simulink model "Digitizing_3delays_1us_pi_wPi2"  (R2014a)
settings: Solver=FixedStepDiscrete  StartTime=0.0  StopTime=0.0  FixedStep=1  RelTol=1e-3
undefined symbols (not defined in the file): inputPulse
libraries: opticalComponentLibrary x23
settings Model: Creator=Nithya Menon  LastModifiedBy=Alexander

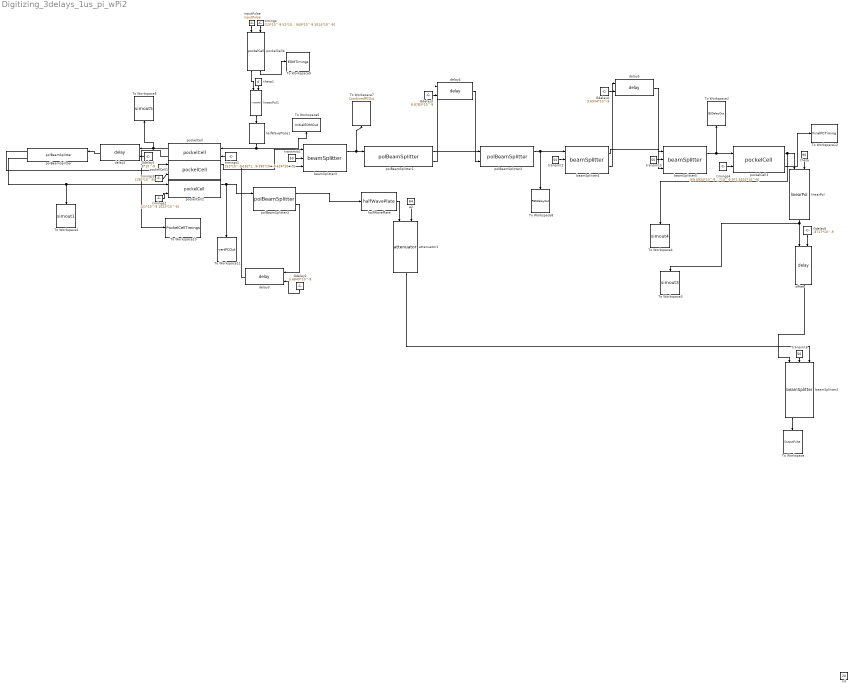
== system Digitizing_3delays_1us_pi_wPi2 ==
  Gdelay1 : Constant  Value=8*10^-9
  Gdelay2 : Constant  Value=5.6849*10^-9
  Gdelay3 : Constant  Value=8.8783*10^-9
  Gdelay4 : Constant  Value=9.6934*10^-9
  Gdelay5 : Constant  Value=.8717*10^-9
  To Workspace : ToWorkspace  VariableName=OutputPulse  SampleTime=-1
  To Workspace1 : ToWorkspace  VariableName=simout1  SampleTime=-1
  To Workspace10 : ToWorkspace  VariableName=PockelCellTimings  SampleTime=-1
  To Workspace11 : ToWorkspace  VariableName=vertPCOut  SampleTime=-1
  To Workspace12 : ToWorkspace  VariableName=FinalPCTiming  SampleTime=-1
  To Workspace2 : ToWorkspace  VariableName=BSDelayOut  SampleTime=-1
  To Workspace3 : ToWorkspace  VariableName=simout3  SampleTime=-1
  To Workspace4 : ToWorkspace  VariableName=simout4  SampleTime=-1
  To Workspace5 : ToWorkspace  VariableName=simout5  SampleTime=-1
  To Workspace6 : ToWorkspace  VariableName=InitialEOMOut  SampleTime=-1
  To Workspace7 : ToWorkspace  VariableName=CombinedPCOut  SampleTime=-1
  To Workspace8 : ToWorkspace  VariableName=PBSDelayOut  SampleTime=-1
  To Workspace9 : ToWorkspace  VariableName=EOMTimings  SampleTime=-1
  a2 : Constant  Value=64
  attenuator1 : opticalComponentLibrary/attenuator
  beamSplitter{2..5} (4 alike) : opticalComponentLibrary/beamSplitter
  delay{2..5} (4 alike) : opticalComponentLibrary/delay
  halfWavePlate : opticalComponentLibrary/halfWavePlate
  halfWavePlate1 : opticalComponentLibrary/halfWavePlate
  inputPulse : Constant  Value=inputPulse
  linearPol : opticalComponentLibrary/linearPol
  linearPol1 : opticalComponentLibrary/linearPol
  n3 : Constant  Value=20
  offset : opticalComponentLibrary/delay
  pockelCell{,1..4} (5 alike) : opticalComponentLibrary/pockelCell
  polBeamSplitter{,1..3} (4 alike) : opticalComponentLibrary/polBeamSplitter
  theta : Constant  Value=90
  theta1 : Constant  Value=0
  timings : Constant  Value="[13*10^-9 52*10^-9 182*10^-9  390*10^-9 624*10^-9 819*10^-9 949*10^-9 1014*10^-9]"
  timings1 : Constant  Value=[52*10^-9 182*10^-9 390*10^-9 624*10^-9]
  timings2 : Constant  Value=[21*10^-9 1022*10^-9]
  timings3 : Constant  Value=[190*10^-9]
  timings4 : Constant  Value=[69.6934*10^-9 198.8783*10^-9 407.6934*10^-9 632*10^-9 851.2566*10^-9 971.5632*10^-9]
  transmit{2..4,6} (4 alike) : Constant  Value=50
  wires:
  inputPulse/1 -> pockelCell4/1
  timings/1 -> pockelCell4/2
  pockelCell/1 -> To Workspace5/1, delay2/1
  Gdelay1/1 -> delay2/2
  delay2/1 -> polBeamSplitter/1
  polBeamSplitter/1 -> pockelCell1/1
  polBeamSplitter/2 -> To Workspace1/1, pockelCell2/1
  Gdelay2/1 -> delay3/2
  timings1/1 -> pockelCell/2
  timings2/1 -> pockelCell2/2
  timings3/1 -> pockelCell1/2
  polBeamSplitter1/1 -> polBeamSplitter2/1
  polBeamSplitter1/2 -> delay4/1
  Gdelay3/1 -> delay4/2
  delay4/1 -> polBeamSplitter2/2
  transmit2/1 -> beamSplitter4/2
  transmit3/1 -> beamSplitter5/2
  polBeamSplitter2/1 -> To Workspace8/1, beamSplitter4/1
  beamSplitter4/1 -> beamSplitter5/1
  Gdelay4/1 -> delay5/2
  beamSplitter4/2 -> delay5/1
  delay5/1 -> beamSplitter5/3
  timings4/1 -> pockelCell3/2
  pockelCell3/1 -> linearPol/1, To Workspace4/1
  transmit4/1 -> beamSplitter3/2
  pockelCell1/1 -> beamSplitter3/1
  theta/1 -> linearPol/2
  pockelCell2/1 -> To Workspace11/1, polBeamSplitter3/1
  polBeamSplitter3/2 -> delay3/1
  delay3/1 -> beamSplitter3/3
  halfWavePlate/1 -> attenuator1/1
  a2/1 -> attenuator1/2
  beamSplitter2/1 -> To Workspace/1
  attenuator1/1 -> beamSplitter2/3
  transmit6/1 -> beamSplitter2/2
  polBeamSplitter3/1 -> halfWavePlate/1
  beamSplitter3/1 -> polBeamSplitter1/1, To Workspace7/1
  Gdelay5/1 -> offset/2
  linearPol/1 -> To Workspace3/1, offset/1
  beamSplitter5/1 -> pockelCell3/1, To Workspace2/1
  pockelCell4/1 -> linearPol1/1
  theta1/1 -> linearPol1/2
  linearPol1/1 -> halfWavePlate1/1
  halfWavePlate1/1 -> To Workspace6/1, pockelCell/1
  offset/1 -> beamSplitter2/1
  pockelCell4/2 -> To Workspace9/1
  pockelCell/2 -> To Workspace10/1
  pockelCell3/2 -> To Workspace12/1
